simulink model "auto_climatecontrol"  (Simulink 6.0)
settings: Solver=ode45  StartTime=0.0  StopTime=1000.0  RelTol=1e-3
libraries: simulink x2
settings Model: Creator=The MathWorks Inc.  LastModifiedBy=batserve  ExtModeAutoUpdateStatusClock=off
settings DataIOCC: SignalLoggingName=sigsOut
settings OptimizationCC: BooleanDataType=off
settings DebuggingCC: CheckExecutionContextPreStartOutputMsg=on  CheckExecutionContextRuntimeOutputMsg=on  SolverPrmCheckMsg=none
settings HardwareCC: TargetUnknown=on

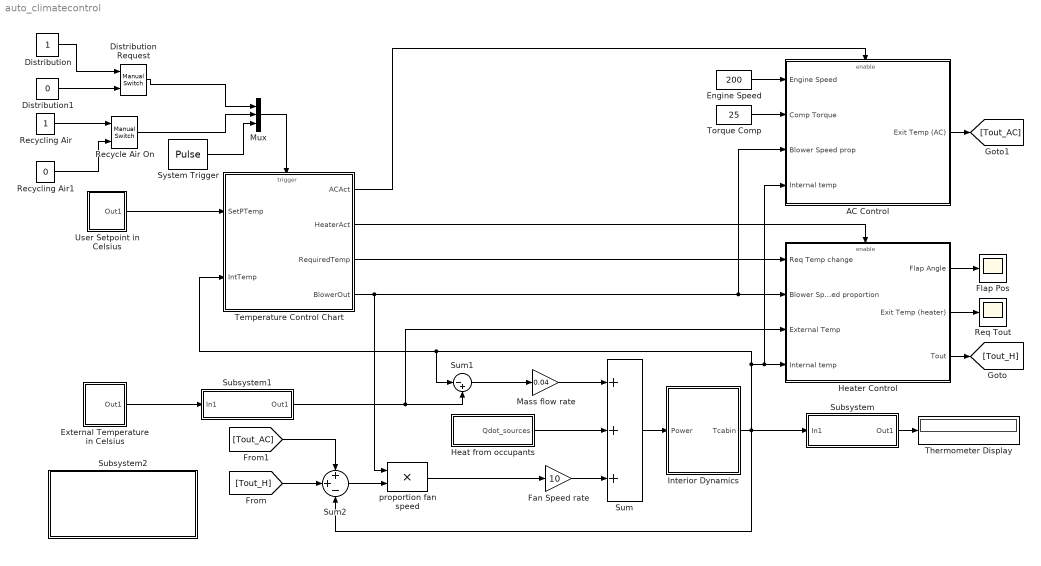
== system auto_climatecontrol ==
  AC Control : Subsystem  TreatAsAtomicUnit=on  PropExecContextAcrossSSBoundary=on
  "Distribution " : Constant
  Distribution Request : simulink/Signal Routing/Manual Switch  sw=0  action=0
  "Distribution1 " : Constant  Value=0
  Engine Speed : Constant  Value=200
  External Temperature in Celsius : Subsystem  PropExecContextAcrossSSBoundary=on  mask(variable){x=18}
      mask prompts: x "Enter the external temperature"
      mask init:
      | set_param('auto_climatecontrol/External Temperature in Celsius/External Temp','Value',num2str(x))
      | external_temp_limit1
      mask Display: disp(x);
  Fan Speed rate : Gain  Gain=10  SaturateOnIntegerOverflow=on
  Flap Pos : Scope
      settings: YMin=41.175  YMax=41.22
  Heat from occupants : Subsystem  PropExecContextAcrossSSBoundary=on  mask(Heat from occupants){N=1}
      mask prompts: N "Number of occupants:"
      settings: AttributesFormatString=No. of occupants: %<N>
      mask Display: disp('Heat Sources')
  Heater Control : Subsystem  TreatAsAtomicUnit=on  PropExecContextAcrossSSBoundary=on
  Interior Dynamics : Subsystem  PropExecContextAcrossSSBoundary=on
      mask Type: Vehicle Cabin Dynamics
      mask Display: image(imread('car_int.jpg'))
  Mass flow rate : Gain  Gain=0.04  SaturateOnIntegerOverflow=on
  Mux : Mux  Inputs=3
  Recycle Air On : simulink/Signal Routing/Manual Switch  sw=0  action=0
  Recycling Air : Constant
  Recycling Air1 : Constant  Value=0
  Req Tout : Scope
      settings: YMin=41.175  YMax=41.22
  Subsystem : Subsystem  PropExecContextAcrossSSBoundary=on
      mask Display: disp('Kelvin to Celsius')
  Subsystem1 : Subsystem  PropExecContextAcrossSSBoundary=on
      mask Display: disp('Celsius to Kelvin')
  Subsystem2 : Subsystem  Orientation=left  PropExecContextAcrossSSBoundary=on
      mask init:
      | % t1=matlabroot;
      | %cd(t1)
      | %test123=which('docCC_file.html','-all');
      | %web(char(test123));
      settings: AttributesFormatString=\n
      settings: OpenFcn=|
      | docfile=which('auto_climatecontrol.html','-all');
      | web(char(docfile));
      mask Display: disp('Double click\nhere for\n Model Information')
  Sum : Sum  Inputs=+++  SaturateOnIntegerOverflow=on  InputSameDT=on
  Sum1 : Sum  Inputs=|-+  SaturateOnIntegerOverflow=on  InputSameDT=on
  Sum2 : Sum  Inputs=++-  SaturateOnIntegerOverflow=on  InputSameDT=on
  System Trigger : DiscretePulseGenerator  PulseType=Time based  Period=1/60  PulseWidth=50
  Temperature Control Chart : Stateflow chart  TreatAsAtomicUnit=on  PropExecContextAcrossSSBoundary=on
  Thermometer Display : Display
  Torque Comp : Constant  Value=25
  User Setpoint in Celsius : Subsystem  PropExecContextAcrossSSBoundary=on  mask{USet=9}
      mask prompts: USet "Enter the Temperature you require"
      mask init:
      | set_param('auto_climatecontrol/User Setpoint in Celsius/User Setpoint','Value',num2str(USet))
      mask Display: disp(num2str(USet))
  proportion fan speed : Product  SaturateOnIntegerOverflow=on  InputSameDT=on
  wires:
  Distribution Request/1 -> Mux/1
  "Distribution "/1 -> Distribution Request/1
  "Distribution1 "/1 -> Distribution Request/2
  Recycling Air1/1 -> Recycle Air On/2
  User Setpoint in Celsius/1(Out1) -> Temperature Control Chart/1(SetPTemp)
  Recycling Air/1 -> Recycle Air On/1
  Recycle Air On/1 -> Mux/2
  System Trigger/1 -> Mux/3
  Interior Dynamics/1("Tcabin ") -> AC Control/4(Internal temp), Heater Control/4(Internal temp), Temperature Control Chart/2(IntTemp), Sum1/1, Sum2/3, Subsystem/1(In1)
  Subsystem/1(Out1) -> Thermometer Display/1
  Heat from occupants/1(Qdot_sources) -> Sum/2
  External Temperature in Celsius/1(Out1) -> Subsystem1/1(In1)
  Mass flow rate/1 -> Sum/1
  Sum1/1 -> Mass flow rate/1
  Subsystem1/1(Out1) -> Heater Control/3(External Temp), Sum1/2
  Fan Speed rate/1 -> Sum/3
  Sum2/1 -> proportion fan speed/2
  Temperature Control Chart/4(BlowerOut) -> AC Control/3(Blower Speed prop), Heater Control/2(Blower Speed proportion), proportion fan speed/1
  proportion fan speed/1 -> Fan Speed rate/1
  Temperature Control Chart/2(HeaterAct) -> Heater Control/Enable
  Heater Control/1(Flap Angle) -> Flap Pos/1
  Heater Control/2(Exit Temp (heater)) -> Req Tout/1
  Heater Control/3(Tout) -> [Tout_H]
  [Tout_H] -> Sum2/2
  Temperature Control Chart/1(ACAct) -> AC Control/Enable
  [Tout_AC] -> Sum2/1
  Torque Comp/1 -> AC Control/2(Comp Torque)
  Temperature Control Chart/3(RequiredTemp) -> Heater Control/1(Req Temp change)
  AC Control/1(Exit Temp (AC)) -> [Tout_AC]
  Engine Speed/1 -> AC Control/1(Engine Speed)
  Mux/1 -> Temperature Control Chart/Trigger
  Sum/1 -> Interior Dynamics/1(Power)

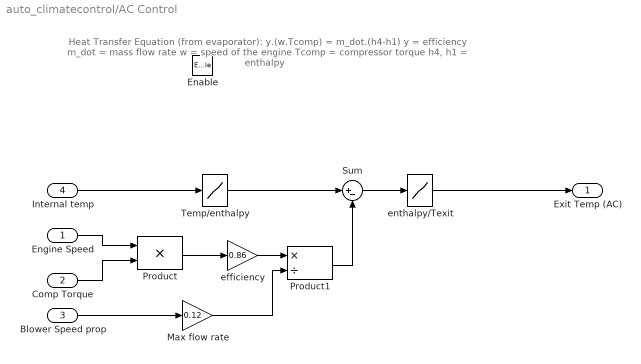
== system auto_climatecontrol/AC Control ==
  note: Heat Transfer Equation (from evaporator):
      |
      | y.(w.Tcomp) = m_dot.(h4-h1)
      |
      | y = efficiency
      | m_dot = mass flow rate
      | w = speed of the engine
      | Tcomp = compressor torque
      | h4, h1 = enthalpy
  Engine Speed : Inport  Port=1  LatchInput=off
  Comp Torque : Inport  Port=2  LatchInput=off
  Blower Speed prop : Inport  Port=3  LatchInput=off
  Internal temp : Inport  Port=4  LatchInput=off
  Enable : EnablePort  StatesWhenEnabling=reset  ZeroCross=off
  Max flow rate : Gain  Gain=0.12  SaturateOnIntegerOverflow=on
  Product : Product  SaturateOnIntegerOverflow=on  InputSameDT=on
  Product1 : Product  Inputs=*/  SaturateOnIntegerOverflow=on  InputSameDT=on
  Sum : Sum  Inputs=|+-  SaturateOnIntegerOverflow=on  InputSameDT=on
  Temp/enthalpy : Lookup  DialogController=Simulink.DDGSource  InputValues=[220 230 240 250 260 270 280 285 290 295 300 305 310 315 320]  OutputValues=[219.97 230.02 240.02 250.05 260.09 270.11 280.13 285.14 290.16 295.17 300.19 305.22 310.24 315.27 320.29]  SaturateOnIntegerOverflow=on
  efficiency : Gain  Gain=0.86  SaturateOnIntegerOverflow=on
  enthalpy/Texit : Lookup  DialogController=Simulink.DDGSource  InputValues=[ 219.97 230.02 240.02 250.05 260.09 270.11 280.13 285.14 290.16 295.17 300.19 305.22 310.24 315.27 320.29]  OutputValues=[220 230 240 250 260 270 280 285 290 295 300 305 310 315 320]  SaturateOnIntegerOverflow=on
  Exit Temp (AC) : Outport  OutputWhenDisabled=reset  InitialOutput=0
  wires:
  Sum/1 -> enthalpy/Texit/1
  Product1/1 -> Sum/2
  Temp/enthalpy/1 -> Sum/1
  Internal temp/1 -> Temp/enthalpy/1
  Max flow rate/1 -> Product1/2
  Blower Speed prop/1 -> Max flow rate/1
  efficiency/1 -> Product1/1
  Product/1 -> efficiency/1
  Comp Torque/1 -> Product/2
  Engine Speed/1 -> Product/1
  enthalpy/Texit/1 -> Exit Temp (AC)/1

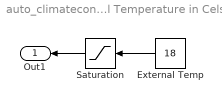
== system auto_climatecontrol/External Temperature in Celsius ==
  External Temp : Constant  Orientation=left  Value=18
  Saturation : Saturate  Orientation=left  UpperLimit=100  LowerLimit=-99
  Out1 : Outport  Orientation=left
  wires:
  External Temp/1 -> Saturation/1
  Saturation/1 -> Out1/1

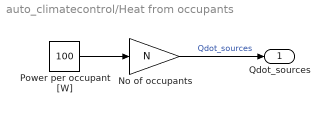
== system auto_climatecontrol/Heat from occupants ==
  No of occupants : Gain  Gain=N  SaturateOnIntegerOverflow=on
  Power per occupant [W] : Constant  Value=100
  Qdot_sources : Outport
  wires:
  Power per occupant [W]/1 -> No of occupants/1
  No of occupants/1 -> Qdot_sources/1  "Qdot_sources"

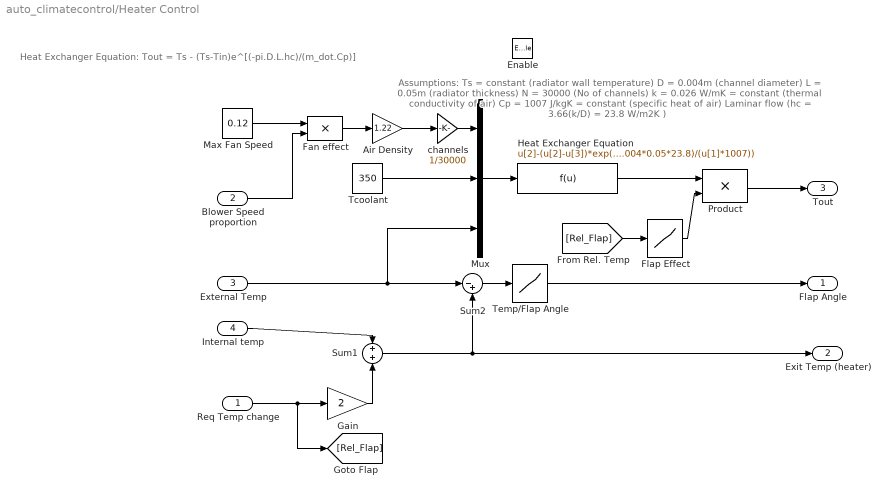
== system auto_climatecontrol/Heater Control ==
  note: Assumptions:
      | Ts = constant (radiator wall temperature)
      | D = 0.004m (channel diameter)
      | L = 0.05m (radiator thickness)
      | N = 30000 (No of channels)
      |
      | k = 0.026 W/mK = constant (thermal conductivity of air)
      | Cp = 1007 J/kgK = constant (specific heat of air)
      | Laminar flow (hc = 3.66(k/D) = 23.8 W/m2K )
  note: Heat Exchanger Equation:
      | Tout = Ts - (Ts-Tin)e^[(-pi.D.L.hc)/(m_dot.Cp)]
  Req Temp change : Inport  Port=1  LatchInput=off
  Blower Speed proportion : Inport  Port=2  LatchInput=off
  External Temp : Inport  Port=3  LatchInput=off
  Internal temp : Inport  Port=4  LatchInput=off
  Enable : EnablePort  StatesWhenEnabling=reset  ZeroCross=off
  Air Density : Gain  Gain=1.22  SaturateOnIntegerOverflow=on
  Fan effect : Product  SaturateOnIntegerOverflow=on  InputSameDT=on
  Flap Effect : Lookup  DialogController=Simulink.DDGSource  InputValues="[0 3 5 10 50  90 100 200 ]"  OutputValues="[0 300 100  10 10  10 3 1]"  SaturateOnIntegerOverflow=on
  Gain : Gain  Gain=2  SaturateOnIntegerOverflow=on
  Heat Exchanger Equation : Fcn  Expr=u[2]-(u[2]-u[3])*exp(-(pi*0.004*0.05*23.8)/(u[1]*1007))
  Max Fan Speed : Constant  Value=0.12
  Mux : Mux  Inputs=3
  Product : Product  SaturateOnIntegerOverflow=on  InputSameDT=on
  Sum1 : Sum  SaturateOnIntegerOverflow=on  InputSameDT=on
  Sum2 : Sum  Inputs=|-+  SaturateOnIntegerOverflow=on  InputSameDT=on
  "Tcoolant " : Constant  Value=350
  Temp/Flap Angle : Lookup  DialogController=Simulink.DDGSource  InputValues=[0 10 20 30 40 50 60 75 100 200]  OutputValues=[0 20 30 45 60 75 90 90 90 90]  SaturateOnIntegerOverflow=on
  channels : Gain  Gain=1/30000  SaturateOnIntegerOverflow=on
  Flap Angle : Outport  OutputWhenDisabled=reset  InitialOutput=0
  Exit Temp (heater) : Outport  Port=2  OutputWhenDisabled=reset  InitialOutput=0
  Tout : Outport  Port=3  OutputWhenDisabled=reset  InitialOutput=0
  wires:
  Heat Exchanger Equation/1 -> Product/1
  External Temp/1 -> Mux/3, Sum2/1
  Blower Speed proportion/1 -> Fan effect/2
  Max Fan Speed/1 -> Fan effect/1
  Fan effect/1 -> Air Density/1
  Mux/1 -> Heat Exchanger Equation/1
  Air Density/1 -> channels/1
  channels/1 -> Mux/1
  "Tcoolant "/1 -> Mux/2
  Flap Effect/1 -> Product/2
  Product/1 -> Tout/1
  Temp/Flap Angle/1 -> Flap Angle/1
  Sum2/1 -> Temp/Flap Angle/1
  Internal temp/1 -> Sum1/1
  Gain/1 -> Sum1/2
  Sum1/1 -> Exit Temp (heater)/1, Sum2/2
  Req Temp change/1 -> Gain/1, [Rel_Flap]
  [Rel_Flap] -> Flap Effect/1

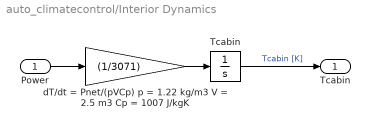
== system auto_climatecontrol/Interior Dynamics ==
  Power : Inport  Port=1  LatchInput=off
  Tcabin : Integrator  InitialCondition=291  ZeroCross=off
  dT/dt = Pnet/(pVCp) p = 1.22 kg/m3 V = 2.5 m3 Cp = 1007 J/kgK : Gain  Gain=(1/3071)  SaturateOnIntegerOverflow=on
  "Tcabin " : Outport
  wires:
  dT/dt = Pnet/(pVCp) p = 1.22 kg/m3 V = 2.5 m3 Cp = 1007 J/kgK/1 -> Tcabin/1
  Power/1 -> dT/dt = Pnet/(pVCp) p = 1.22 kg/m3 V = 2.5 m3 Cp = 1007 J/kgK/1
  Tcabin/1 -> "Tcabin "/1  "Tcabin [K]"

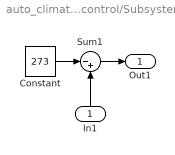
== system auto_climatecontrol/Subsystem ==
  In1 : Inport  Orientation=up  Port=1  LatchInput=off
  Constant : Constant  Value=273
  Sum1 : Sum  Inputs=|-+  SaturateOnIntegerOverflow=on  InputSameDT=on
  Out1 : Outport
  wires:
  Sum1/1 -> Out1/1
  In1/1 -> Sum1/2
  Constant/1 -> Sum1/1

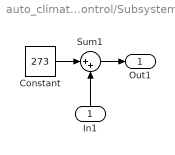
== system auto_climatecontrol/Subsystem1 ==
  In1 : Inport  Orientation=up  Port=1  LatchInput=off
  Constant : Constant  Value=273
  Sum1 : Sum  Inputs=|++  SaturateOnIntegerOverflow=on  InputSameDT=on
  Out1 : Outport
  wires:
  Constant/1 -> Sum1/1
  In1/1 -> Sum1/2
  Sum1/1 -> Out1/1

== system auto_climatecontrol/Subsystem2 ==

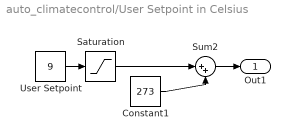
== system auto_climatecontrol/User Setpoint in Celsius ==
  Constant1 : Constant  Value=273
  Saturation : Saturate  UpperLimit=100  LowerLimit=-99
  Sum2 : Sum  Inputs=|++  SaturateOnIntegerOverflow=on  InputSameDT=on
  User Setpoint : Constant  Value=9
  Out1 : Outport
  wires:
  Sum2/1 -> Out1/1
  User Setpoint/1 -> Saturation/1
  Constant1/1 -> Sum2/2
  Saturation/1 -> Sum2/1

== stateflow chart Temperature Control Chart ==
  state Blower [parallel]
    during:setpoint_calc();
    state Blower_off
      entry:BlowerOut=0.0;
    state Blower_on
      state Blower_1
        entry:BlowerOut=0.2;
      state Blower_2
        entry:BlowerOut=0.4;
      state Blower_3
        entry:BlowerOut=0.6;
      state Blower_5
        entry:BlowerOut=1.0;
      state Blower_4
        entry:BlowerOut=0.8;
      Blower_on -> Blower_2 : E[!in(Blower_2) && in_temp_range(7,10)]
      Blower_on -> Blower_1 : E[!in(Blower_1) && in_temp_range(1.5,5)]
      Blower_on -> Blower_3 : E[!in(Blower_3) && in_temp_range(12,15)]
      Blower_on -> Blower_4 : E[!in(Blower_4) && in_temp_range(17,20)]
      Blower_on -> Blower_5 : E[!in(Blower_5) && in_temp_range(22,200)]
      (default) -> Blower_1
    state b = in_temp_range(minTemp,maxTemp) [function]
      (default) -> (junction 26) : {b = (absTempDiff>minTemp) &&  ...
          |         (absTempDiff<maxTemp);}
    state setpoint_calc() [function]
      (default) -> (junction 27) : {RequiredTemp = SetPTemp-IntTemp;}
      (junction 27) -> (junction 24) : [RequiredTemp<0.0]
          | {absTempDiff = -RequiredTemp;}
      (junction 27) -> (junction 25) : {absTempDiff = RequiredTemp;}
    (default) -> Blower_off
    Blower_on -> Blower_off : E[absTempDiff>203 || absTempDiff<=0.5]
    Blower_off -> Blower_on : E[in_temp_range(.5,203)]
  state Recyc_Air [parallel]
    state Recyc_on
    state Recyc_off
    Recyc_on -> Recyc_off : en(AirDist.Defrost)
    (default) -> Recyc_on
    Recyc_on -> Recyc_off : RecycReq
    Recyc_off -> Recyc_on : RecycReq
  state Heater_AC [parallel]
    state H_offAC_off
    state HeaterAct
    state ACAct
    ACAct -> H_offAC_off : E[SetPTemp-IntTemp>=-0.5]
    H_offAC_off -> ACAct : E[SetPTemp-IntTemp<-0.5]
    H_offAC_off -> HeaterAct : E[SetPTemp-IntTemp>0.5]
    HeaterAct -> H_offAC_off : E[SetPTemp-IntTemp<=0.5]
    (default) -> H_offAC_off
  state AirDist [parallel]
    state Face
    state Feet
    state Defrost
    (default) -> Face
    Defrost -> Face : DistReq
    Feet -> Defrost : DistReq
    Face -> Feet : DistReq
  data: minTemp function_input double; b function_output boolean; maxTemp function_input double; ACAct output State; SetPTemp input double; IntTemp input double; HeaterAct output State; RequiredTemp output double; BlowerOut output double; absTempDiff local double
  events: DistReq input EITHER_EDGE_EVENT; RecycReq input EITHER_EDGE_EVENT; E input EITHER_EDGE_EVENT
